simulink model "equation_motion"  (R2015b)
settings: Solver=VariableStepAuto  StartTime=0.0  StopTime=10.0  RelTol=1e-3
values from neighbouring files (symbols this model uses):
  Velocity = vel    [RHC_opt.m]    (also in RHC_opt_mod_algo.m; search_and_coverage.m = sqrt(2*Weight/(rho*W_area)*(1/CL)); search_and_coverage_multiple_turn_durations.m = sqrt(2*Weight/(rho*W_area)*(1/CL)); search_and_coverage_time_constraint.m = sqrt(2*Weight/(rho*W_area)*(1/CL)))
settings Model: Creator=gggramajo  LastModifiedBy=gggramajo

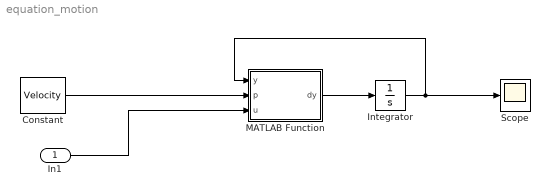
== system equation_motion ==
  In1 : Inport
  Constant : Constant  Value=Velocity
  Integrator : Integrator
  MATLAB Function : MATLAB Function  TreatAsAtomicUnit=on
  Scope : Scope
  wires:
  Integrator/1 -> MATLAB Function/1(y), Scope/1
  MATLAB Function/1(dy) -> Integrator/1
  Constant/1 -> MATLAB Function/2(p)
  In1/1 -> MATLAB Function/3(u)

== matlab function equation_motion/MATLAB Function ==
  data: y input; p input; dy output; u input
function dy = fcn(y,p,u)
dy=zeros(3,1);
dy(1)=p*cos(y(3));
dy(2)=p*sin(y(3));
dy(3)=u;
